simulink model "SILTest"  (R2018b)
settings: Solver=FixedStepDiscrete  StartTime=0.0  StopTime=10.0  FixedStep=0.1  RelTol=1e-3
values from neighbouring files (symbols this model uses):
  Tbl = createCfsTbl(TblVals, 'Tbl')    [init.m]
libraries: cfs_library x4
settings Model: Creator=slentine  LastModifiedBy=slentine
settings OptimizationCC: DefaultParameterBehavior=Inlined  EnhancedBackFolding=on  PassReuseOutputArgsAs=Individual arguments  OptimizeBlockOrder=speed  DifferentSizesBufferReuse=on  OptimizationCustomize=off
settings DebuggingCC: ParameterTunabilityLossMsg=error
settings SFSimCC: MATLABDynamicMemAlloc=off
settings RTWCC: SystemTargetFile=cfs_ert.tlc  GenCodeOnly=on  TemplateMakefile=ert_default_tmf  Description=NASA CFS Target File  GenerateReport=on  IncludeHyperlinkInReport=on  LaunchReport=on  GenerateTraceInfo=on  GenerateTraceReport=on  GenerateTraceReportSl=on  GenerateTraceReportSf=on  GenerateTraceReportEml=on
settings CodeAppCC: ForceParamTrailComments=on  IgnoreCustomStorageClasses=off  OperatorAnnotations=on  SimulinkDataObjDesc=on  SFDataObjDesc=on  InsertBlockDesc=on
settings STFCustomTargetCC: TargetLangStandard=C99 (ISO)  MultiwordLength=256  CombineOutputUpdateFcns=on  ERTCustomFileBanners=on  SupportContinuousTime=off  SupportNonInlinedSFcns=off  RemoveResetFunc=on  MATLABClassNameForMDSCustomization=Simulink.SoftwareTarget.ERTCustomization  UseToolchainInfoCompliant=on  SystemTargetFile=cfs_ert.tlc
settings ERTTargetCC: TargetLangStandard=C99 (ISO)  ParMdlRefBuildCompliant=off  CompOptLevelCompliant=off  ConcurrentExecutionCompliant=off  ModelStepFunctionPrototypeControlCompliant=off  CPPClassGenCompliant=off  InlinedParameterPlacement=NonHierarchical  ERTCustomFileTemplate=cfs_interface.tlc

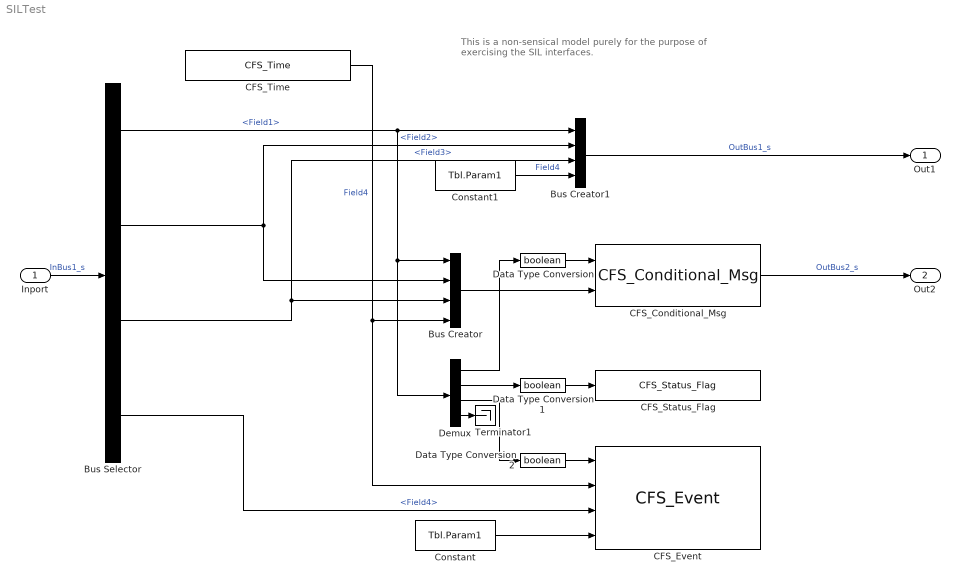
== system SILTest ==
  note: This is a non-sensical model purely for the purpose
      | of exercising the SIL interfaces.
  Inport : Inport  OutDataTypeStr=Bus: InBus_1_b  Interpolate=off  BusOutputAsStruct=on
  Bus Creator : BusCreator  Inputs=4  OutDataTypeStr=Bus: OutBus_2_b  NonVirtualBus=on
  Bus Creator1 : BusCreator  Inputs=4  OutDataTypeStr=Bus: OutBus_1_b  NonVirtualBus=on
  Bus Selector : BusSelector  OutputSignals=Field1,Field2,Field3,Field4
  CFS_Conditional_Msg : cfs_library/CFS_Conditional_Msg  bus_name=[]  bus_type=Bus: OutBus_2_b  block_sid=[]
      settings: SourceProductName=CFS Blockset
  CFS_Event : cfs_library/CFS_Event  event_id=14  event_type=uint16(12)  event_mask=0  string_data='%f %e %e '  fmt_string=uint8(['Loc: %s, %f %e %e ' 0])  num_data_ports=3  block_sid=0
      settings: SourceProductName=CFS Blockset
  CFS_Status_Flag : cfs_library/CFS_Status_Flag  fdc_id=14  block_sid=0
      settings: SourceProductName=CFS Blockset
  CFS_Time : cfs_library/CFS_Time  SFunctionSpec=double y1 = get_gps(double p1)  SParameter1=0.0  SParameter2=0.1
      settings: SourceProductName=CFS Blockset
  Constant : Constant  Value=Tbl.Param1
  Constant1 : Constant  Value=Tbl.Param1
  Data Type Conversion : DataTypeConversion  OutDataTypeStr=boolean
  Data Type Conversion1 : DataTypeConversion  OutDataTypeStr=boolean
  Data Type Conversion2 : DataTypeConversion  OutDataTypeStr=boolean
  Demux : Demux  Outputs=[1 1 1 5]
  Terminator1 : Terminator
  Out1 : Outport  OutDataTypeStr=Bus: OutBus_1_b
  Out2 : Outport  Port=2  OutDataTypeStr=Bus: OutBus_2_b
  wires:
  CFS_Conditional_Msg/1 -> Out2/1  "OutBus2_s"
  Bus Creator/1 -> CFS_Conditional_Msg/2
  Bus Creator1/1 -> Out1/1  "OutBus1_s"
  Inport/1 -> Bus Selector/1  "InBus1_s"
  CFS_Time/1 -> Bus Creator/4, CFS_Event/2  "Field4"
  Bus Selector/1 -> Bus Creator/1, Demux/1, Bus Creator1/1  "<Field1>"
  Demux/1 -> Data Type Conversion/1
  Demux/2 -> Data Type Conversion1/1
  Demux/3 -> Data Type Conversion2/1
  Bus Selector/2 -> Bus Creator1/2, Bus Creator/2  "<Field2>"
  Bus Selector/3 -> Bus Creator/3, Bus Creator1/3  "<Field3>"
  Bus Selector/4 -> CFS_Event/3  "<Field4>"
  Demux/4 -> Terminator1/1
  Data Type Conversion/1 -> CFS_Conditional_Msg/1
  Data Type Conversion1/1 -> CFS_Status_Flag/1
  Data Type Conversion2/1 -> CFS_Event/1
  Constant/1 -> CFS_Event/4
  Constant1/1 -> Bus Creator1/4  "Field4"
